simulink model "FeedbackLinearize"  (R2013a)
settings: Solver=ode45  StartTime=0.0  StopTime=10.0  RelTol=1e-3
settings Model: Creator=Walter  LastModifiedBy=daqing_yi
settings DataIOCC: SignalLoggingSaveFormat=ModelDataLogs
settings DebuggingCC: MultiTaskDSMMsg=warning  MultiTaskCondExecSysMsg=none  StateNameClashWarn=none  StrictBusMsg=None
settings RTWCC: IncludeERTFirstTime=on

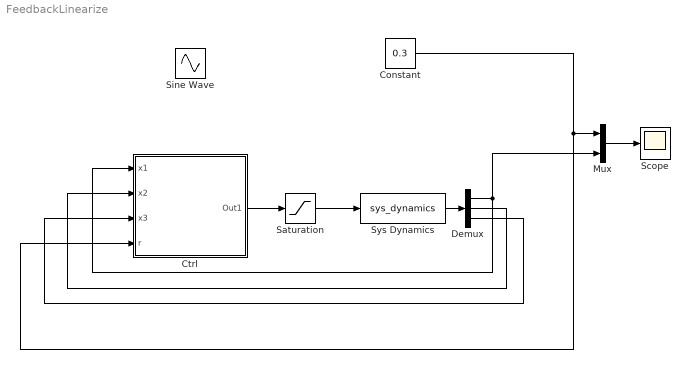
== system FeedbackLinearize ==
  Constant : Constant  Value=0.3
  "Ctrl " : Subsystem
  Demux : Demux  Outputs=3
  Mux : Mux  Inputs=2
  Saturation : Saturate  UpperLimit=5  LowerLimit=-5
  Scope : Scope
      settings: YMin=-3.25e+22  YMax=2.5e+21
  Sine Wave : Sin  Amplitude=0.01  Bias=0.05  SampleTime=0
  Sys Dynamics : S-Function  FunctionName=sys_dynamics  EnableBusSupport=off
  wires:
  Sys Dynamics/1 -> Demux/1
  Constant/1 -> "Ctrl "/4(r), Mux/1
  Demux/2 -> "Ctrl "/2(x2)
  Demux/3 -> "Ctrl "/3(x3)
  Mux/1 -> Scope/1
  Demux/1 -> "Ctrl "/1(x1), Mux/2
  Saturation/1 -> Sys Dynamics/1
  "Ctrl "/1(Out1) -> Saturation/1

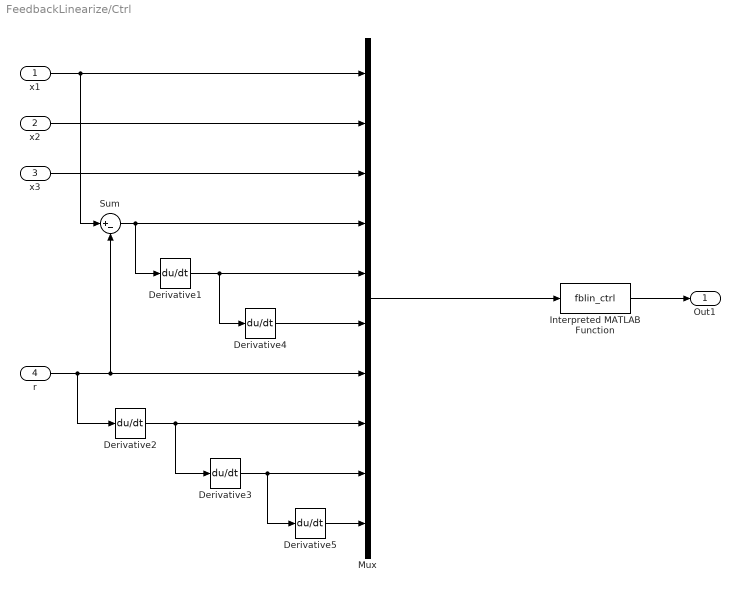
== system FeedbackLinearize/Ctrl  ==
  x1 : Inport
  x2 : Inport  Port=2
  x3 : Inport  Port=3
  r : Inport  Port=4
  Derivative{1..5} (5 alike) : Derivative
  Interpreted MATLAB Function : MATLABFcn  MATLABFcn=fblin_ctrl
  Mux : Mux  Inputs=10
  Sum : Sum  Inputs=|+-
  Out1 : Outport
  wires:
  x3/1 -> Mux/3
  x2/1 -> Mux/2
  Interpreted MATLAB Function/1 -> Out1/1
  x1/1 -> Sum/1, Mux/1
  r/1 -> Sum/2, Mux/7, Derivative2/1
  Derivative3/1 -> Derivative5/1, Mux/9
  Derivative2/1 -> Derivative3/1, Mux/8
  Mux/1 -> Interpreted MATLAB Function/1
  Sum/1 -> Derivative1/1, Mux/4
  Derivative1/1 -> Derivative4/1, Mux/5
  Derivative4/1 -> Mux/6
  Derivative5/1 -> Mux/10
